simulink model "MF_FiO2"  (R2022a)
settings: Solver=FixedStepAuto  StartTime=0.0  StopTime=30.0  RelTol=1e-3  EnableMultiTasking=on
libraries: simulink x4, mbedblockslib x3
settings Model: ExtModeTrigDuration=10  Creator=smith  LastModifiedBy=smith
settings OptimizationCC: EnhancedBackFolding=on  PassReuseOutputArgsAs=Individual arguments  ZeroExternalMemoryAtStartup=off  ZeroInternalMemoryAtStartup=off  MaxStackSize=64  OptimizeBlockOrder=speed  DifferentSizesBufferReuse=on  OptimizationCustomize=off  EfficientTunableParamExpr=on
settings DebuggingCC: ParameterTunabilityLossMsg=error
settings HardwareCC: ProdBitPerPointer=32  ProdBitPerSizeT=32  ProdBitPerPtrDiffT=32  ProdLargestAtomicInteger=Long  ProdLargestAtomicFloat=Double  ProdWordSize=32  ProdLongLongMode=on  ProdHWDeviceType=ARM Compatible->ARM Cortex
settings SFSimCC: MATLABDynamicMemAlloc=off
settings RTWCC: SystemTargetFile=ert.tlc  HardwareBoard=STM32 Nucleo L476RG  TemplateMakefile=ert_default_tmf  Toolchain=GNU Tools for ARM Embedded Processors
settings CodeAppCC: ForceParamTrailComments=on  IgnoreCustomStorageClasses=off  OperatorAnnotations=on  SimulinkDataObjDesc=on  SFDataObjDesc=on  InsertBlockDesc=on
settings ERTTargetCC: SupportContinuousTime=on  ExtModeTransport=3  ExtModeStaticAlloc=on  ExtModeStaticAllocSize=2000  ExtModeMexFile=ext_xcp  ExtModeIntrfLevel=Level2 - Open

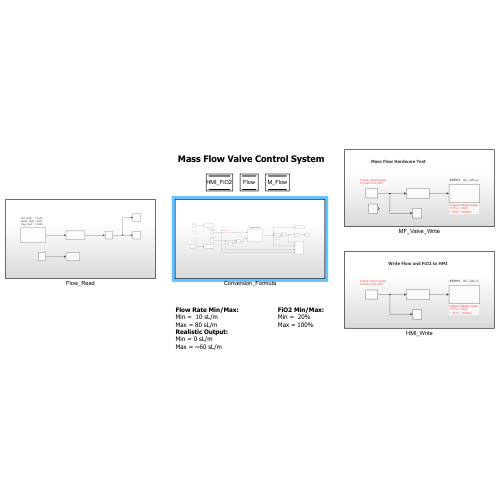
[thumbnail: Simulink's stored preview of the top-level diagram]
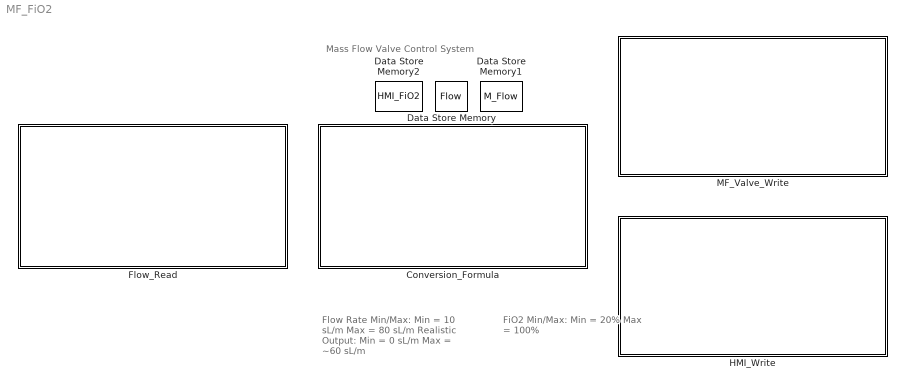
== system MF_FiO2 ==
  note: Flow Rate Min/Max:
      | Min = 10 sL/m
      | Max = 80 sL/m
      | Realistic Output:
      | Min = 0 sL/m
      | Max = ~60 sL/m
  note: Mass Flow Valve Control System
  note: FiO2 Min/Max:
      | Min = 20%
      | Max = 100%
  Conversion_Formula : Subsystem
  Data Store Memory : DataStoreMemory  DataStoreName=Flow  WriteAfterWriteMsg=warning  ShowAdditionalParam=off
  Data Store Memory1 : DataStoreMemory  DataStoreName=M_Flow  WriteAfterWriteMsg=warning  ShowAdditionalParam=off
  Data Store Memory2 : DataStoreMemory  DataStoreName=HMI_FiO2  WriteAfterWriteMsg=warning  ShowAdditionalParam=off
  Flow_Read : Subsystem
  HMI_Write : Subsystem
  MF_Valve_Write : Subsystem

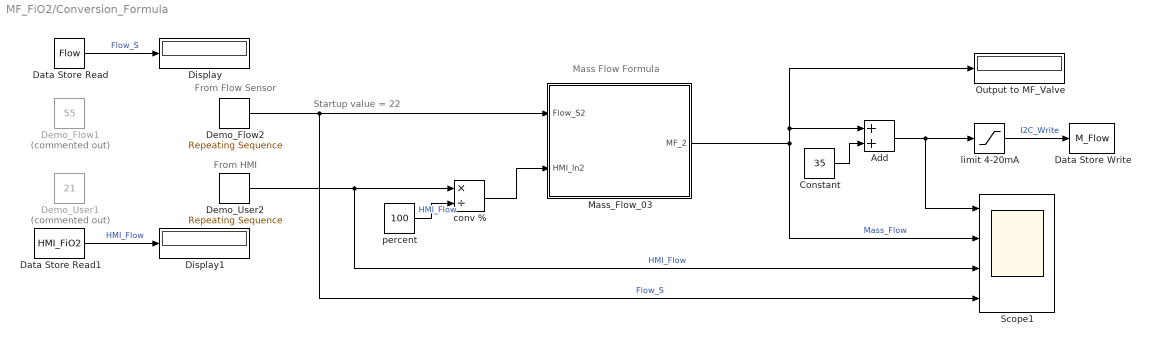
== system MF_FiO2/Conversion_Formula ==
  note: From HMI
  note: From Flow Sensor
  note: Mass Flow Formula
  note: Startup value = 22
  Add : Sum
  Constant : Constant  Value=35
  Data Store Read : DataStoreRead  DataStoreName=Flow  IndexOptions=Index vector (dialog)  Indices=1  OutputSizes=1
  Data Store Read1 : DataStoreRead  DataStoreName=HMI_FiO2  IndexOptions=Index vector (dialog)  Indices=1  OutputSizes=1
  Data Store Write : DataStoreWrite  DataStoreName=M_Flow  IndexOptions=Index vector (dialog)  Indices=1  OutputSizes=1
  Demo_Flow1 : Constant  Commented=on  Value=55
  Demo_Flow2 : simulink/Sources/Repeating Sequence  rep_seq_t=[0 10 10.1 20 20.1 30 30.1 40 40.1]  rep_seq_y=[21 21 35 35 21 21 35 35 21]
  Demo_User1 : Constant  Commented=on  Value=21
  Demo_User2 : simulink/Sources/Repeating Sequence  rep_seq_t=[0 1 1.1 2 2.1 3 3.1 4 4.1]  rep_seq_y=[21 21 65 65 35 35 45 45 20]
  Display : Display
  Display1 : Display
  Mass_Flow_03 : Subsystem
  Output to MF_Valve : Display
  Scope1 : Scope  NumInputPorts=4
  conv % : Product  Inputs=*/
  limit 4-20mA : Saturate  UpperLimit=255  LowerLimit=35
  percent : Constant  Value=100
  wires:
  Data Store Read1/1 -> Display1/1  "HMI_Flow"
  Data Store Read/1 -> Display/1  "Flow_S"
  conv %/1 -> Mass_Flow_03/2(HMI_In2)
  Demo_Flow2/1 -> Scope1/4, Mass_Flow_03/1(Flow_S2)  "Flow_S"
  percent/1 -> conv %/2  "HMI_Flow"
  Demo_User2/1 -> Scope1/3, conv %/1  "HMI_Flow"
  Add/1 -> Scope1/1, limit 4-20mA/1
  Constant/1 -> Add/2
  Mass_Flow_03/1(MF_2) -> Scope1/2, Output to MF_Valve/1, Add/1  "Mass_Flow"
  limit 4-20mA/1 -> Data Store Write/1  "I2C_Write"

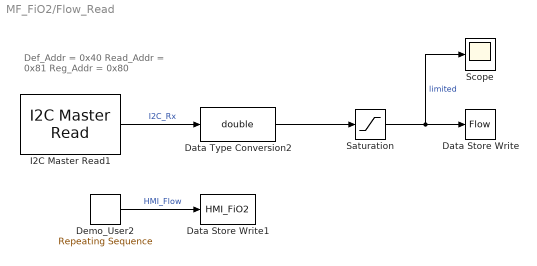
== system MF_FiO2/Flow_Read ==
  note: Def_Addr = 0x40
      | Read_Addr = 0x81
      | Reg_Addr = 0x80
  Data Store Write : DataStoreWrite  DataStoreName=Flow  IndexOptions=Index vector (dialog)  Indices=1  OutputSizes=1
  Data Store Write1 : DataStoreWrite  DataStoreName=HMI_FiO2  IndexOptions=Index vector (dialog)  Indices=1  OutputSizes=1
  Data Type Conversion2 : DataTypeConversion  OutDataTypeStr=double  SaturateOnIntegerOverflow=off  RndMeth=Floor
  Demo_User2 : simulink/Sources/Repeating Sequence  rep_seq_t=[0 1 1.1 2 2.1 3 3.1 4 4.1]  rep_seq_y=[21 21 65 65 35 35 45 45 20]
  I2C Master Read1 : mbedblockslib/I2C Master Read  I2CModule=0  Mode=Master  SlaveAddress=hex2dec('0x11')  SlaveByteOrder=BigEndian  Direction=Receiver  RegisterAddressMode=off  RegisterAddress=uint8(1)  SlaveDataType=uint8  DataLength=1  NoAck=off  RepeatedStart=off  OutputStatus=off  SampleTime=0.1
      settings: SourceProductBaseCode=MICROBIT,NUCLEO,STMICRODIS
  Saturation : Saturate  UpperLimit=255  LowerLimit=-255
  Scope : Scope
  wires:
  Saturation/1 -> Data Store Write/1, Scope/1  "limited"
  I2C Master Read1/1 -> Data Type Conversion2/1  "I2C_Rx"
  Data Type Conversion2/1 -> Saturation/1
  Demo_User2/1 -> Data Store Write1/1  "HMI_Flow"

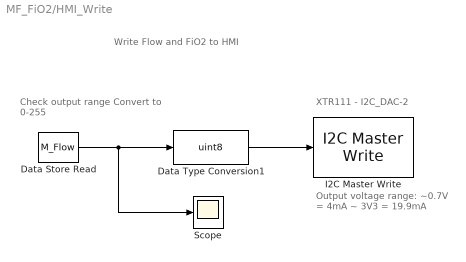
== system MF_FiO2/HMI_Write ==
  note: XTR111 - I2C_DAC-2
  note: Output voltage range:
      | ~0.7V = 4mA
      | ~ 3V3 = 19.9mA
  note: Write Flow and FiO2 to HMI
  note: Check output range
      | Convert to 0-255
  Data Store Read : DataStoreRead  DataStoreName=M_Flow  IndexOptions=Index vector (dialog)  Indices=1  OutputSizes=1
  Data Type Conversion1 : DataTypeConversion  OutDataTypeStr=uint8  SaturateOnIntegerOverflow=off  RndMeth=Floor
  I2C Master Write : mbedblockslib/I2C Master Write  I2CModule=2  Mode=Master  SlaveAddress=uint8(hex2dec('2A'))  SlaveByteOrder=BigEndian  Direction=Transmitter  RegisterAddressMode=on  RegisterAddress=uint8(hex2dec('11'))  SlaveDataType=uint8  DataLength=2  NoAck=off  RepeatedStart=off  OutputStatus=off
      settings: SourceProductBaseCode=MICROBIT,NUCLEO,STMICRODIS
  Scope : Scope
  wires:
  Data Type Conversion1/1 -> I2C Master Write/1
  Data Store Read/1 -> Data Type Conversion1/1, Scope/1

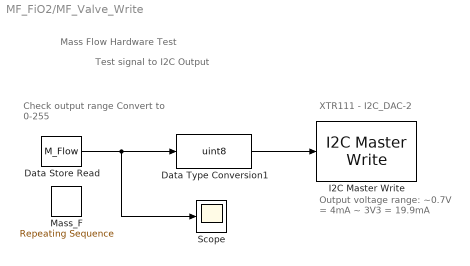
== system MF_FiO2/MF_Valve_Write ==
  note: Check output range
      | Convert to 0-255
  note: Mass Flow Hardware Test
  note: Test signal to I2C Output
  note: Output voltage range:
      | ~0.7V = 4mA
      | ~ 3V3 = 19.9mA
  note: XTR111 - I2C_DAC-2
  Data Store Read : DataStoreRead  DataStoreName=M_Flow  IndexOptions=Index vector (dialog)  Indices=1  OutputSizes=1
  Data Type Conversion1 : DataTypeConversion  OutDataTypeStr=uint8  SaturateOnIntegerOverflow=off  RndMeth=Floor
  I2C Master Write : mbedblockslib/I2C Master Write  I2CModule=2  Mode=Master  SlaveAddress=uint8(hex2dec('2A'))  SlaveByteOrder=BigEndian  Direction=Transmitter  RegisterAddressMode=on  RegisterAddress=uint8(hex2dec('11'))  SlaveDataType=uint8  DataLength=2  NoAck=off  RepeatedStart=off  OutputStatus=off
      settings: SourceProductBaseCode=MICROBIT,NUCLEO,STMICRODIS
  Mass_F : simulink/Sources/Repeating Sequence  rep_seq_t=[0 1 1.1 3 3.1 5 5.1 7 7.1 9]  rep_seq_y=[75 75 120 120 200 200 150 150 75 75]
  Scope : Scope
  wires:
  Data Store Read/1 -> Scope/1, Data Type Conversion1/1
  Data Type Conversion1/1 -> I2C Master Write/1

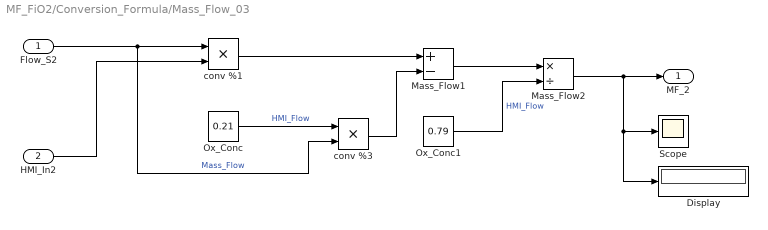
== system MF_FiO2/Conversion_Formula/Mass_Flow_03 ==
  Flow_S2 : Inport
  HMI_In2 : Inport  Port=2
  Display : Display
  Mass_Flow1 : Sum  Inputs=+-
  Mass_Flow2 : Product  Inputs=*/
  Ox_Conc : Constant  Value=0.21
  Ox_Conc1 : Constant  Value=0.79
  Scope : Scope
  conv %1 : Product  Inputs=**
  conv %3 : Product  Inputs=**
  MF_2 : Outport
  wires:
  HMI_In2/1 -> conv %1/2
  Ox_Conc/1 -> conv %3/1  "HMI_Flow"
  conv %3/1 -> Mass_Flow1/2
  Mass_Flow2/1 -> Display/1, Scope/1, MF_2/1
  Mass_Flow1/1 -> Mass_Flow2/1
  Flow_S2/1 -> conv %1/1, conv %3/2  "Mass_Flow"
  Ox_Conc1/1 -> Mass_Flow2/2  "HMI_Flow"
  conv %1/1 -> Mass_Flow1/1
